simulink model "Thruster"  (R2019a)
settings: Solver=VariableStepAuto  StartTime=0.0  StopTime=10.0  RelTol=1e-3
undefined symbols (not defined in the file or in its folder): Force_thruster, GT, uT
libraries: vrlib x1
settings Model: Creator=brice  LastModifiedBy=brice

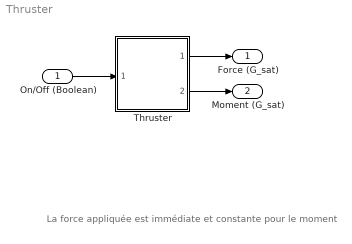
== system Thruster ==
  note: La force appliquée est immédiate et constante pour le moment
  On/Off (Boolean) : Inport
  Thruster : Subsystem
  Force (G_sat) : Outport
  Moment (G_sat) : Outport  Port=2
  wires:
  On/Off (Boolean)/1 -> Thruster/1(On/Off (Boolean))
  Thruster/1(Force (G_sat)) -> Force (G_sat)/1
  Thruster/2(Moment (G_sat)) -> Moment (G_sat)/1

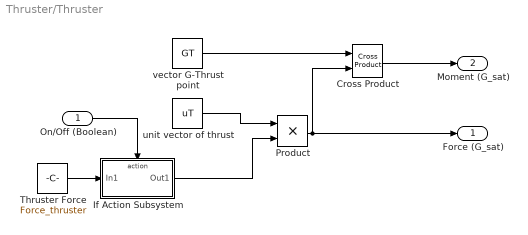
== system Thruster/Thruster ==
  On/Off (Boolean) : Inport
  Cross Product : vrlib/Utilities/Cross Product
      settings: SourceProductName=Simulink
  If Action Subsystem : Subsystem  TreatAsAtomicUnit=on
  Product : Product
  Thruster Force : Constant  Value=Force_thruster
  unit vector of thrust : Constant  Value=uT
  vector G-Thrust point : Constant  Value=GT
  Force (G_sat) : Outport
  Moment (G_sat) : Outport  Port=2
  wires:
  Product/1 -> Force (G_sat)/1, Cross Product/2
  On/Off (Boolean)/1 -> If Action Subsystem/Action
  If Action Subsystem/1(Out1) -> Product/2
  vector G-Thrust point/1 -> Cross Product/1
  unit vector of thrust/1 -> Product/1
  Cross Product/1 -> Moment (G_sat)/1
  Thruster Force/1 -> If Action Subsystem/1(In1)

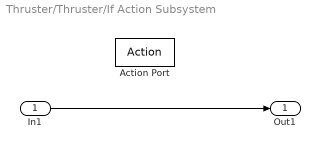
== system Thruster/Thruster/If Action Subsystem ==
  In1 : Inport
  Action Port : ActionPort
  Out1 : Outport  VectorParamsAs1DForOutWhenUnconnected=on
  wires:
  In1/1 -> Out1/1
